simulink subsystem "ACS_Software"  (R2024a)
settings: Solver=VariableStepAuto  StartTime=0.0  StopTime=10.0  RelTol=1e-3
undefined symbols (not defined in the file): epoch, IAU, juliandate, k_Bdot, Kd, km, Kp, m, NoiseStd, s, signQuat, simulator, WMM2020
libraries: sharedtransform x15, simulink_extras x8, aerolibconvert2 x6, matrix_library x5, aerolibutil x5, aerolibtransform2 x2, sharedutil x1, SepehrMILLib x1, aerolibgravity2 x1
(part 2 of 2)

== system ACS_Software/Onboard Model of Environment/Reference Frames Transformations Manager/Quaternion Conditioner3 ==
  Q : Inport  PortDimensions=[4,1]
  Interpreted MATLAB Function : MATLABFcn  MATLABFcn=[u(1),0,0,0;0,u(2),0,0;0,0,u(3),0;0,0,0,u(4)]
  Interpreted MATLAB Function1 : MATLABFcn  MATLABFcn=[u(1),0,0,0;0,u(2),0,0;0,0,u(3),0;0,0,0,u(4)]
  Interpreted MATLAB Function2 : MATLABFcn  MATLABFcn=(u(1)+u(6)+u(11)+u(16))+1.9
  Product : Product
  Product1 : Product
  Sign : Signum
  Sign1 : Signum
  Unit Delay : UnitDelay  InitialCondition=[1;0;0;0]  SampleTime=-1  HasFrameUpgradeWarning=on
  Qc : Outport  PortDimensions=[4,1]
  wires:
  Unit Delay/1 -> Interpreted MATLAB Function1/1
  Interpreted MATLAB Function1/1 -> Product/2
  Q/1 -> Product1/1, Interpreted MATLAB Function/1
  Sign1/1 -> Product1/2
  Product/1 -> Sign/1
  Sign/1 -> Interpreted MATLAB Function2/1
  Interpreted MATLAB Function2/1 -> Sign1/1
  Interpreted MATLAB Function/1 -> Product/1
  Product1/1 -> Unit Delay/1, Qc/1

== system ACS_Software/Onboard Model of Environment/Reference Frames Transformations Manager/Quaternion Conditioner4 ==
  Q : Inport  PortDimensions=[4,1]
  Interpreted MATLAB Function : MATLABFcn  MATLABFcn=[u(1),0,0,0;0,u(2),0,0;0,0,u(3),0;0,0,0,u(4)]
  Interpreted MATLAB Function1 : MATLABFcn  MATLABFcn=[u(1),0,0,0;0,u(2),0,0;0,0,u(3),0;0,0,0,u(4)]
  Interpreted MATLAB Function2 : MATLABFcn  MATLABFcn=(u(1)+u(6)+u(11)+u(16))+1.9
  Product : Product
  Product1 : Product
  Sign : Signum
  Sign1 : Signum
  Unit Delay : UnitDelay  InitialCondition=[1;0;0;0]  SampleTime=-1  HasFrameUpgradeWarning=on
  Qc : Outport  PortDimensions=[4,1]
  wires:
  Product1/1 -> Qc/1, Unit Delay/1
  Interpreted MATLAB Function/1 -> Product/1
  Interpreted MATLAB Function2/1 -> Sign1/1
  Sign/1 -> Interpreted MATLAB Function2/1
  Product/1 -> Sign/1
  Sign1/1 -> Product1/2
  Q/1 -> Interpreted MATLAB Function/1, Product1/1
  Interpreted MATLAB Function1/1 -> Product/2
  Unit Delay/1 -> Interpreted MATLAB Function1/1

== matlab function ACS_Software/Attitude Determination and Estimation Algorithms/Quaternion Conditioner/MATLAB Function ==
  data: Diag_q input; y output
function y = fcn(Diag_q)

y = diag(Diag_q);

== matlab function ACS_Software/Attitude Determination and Estimation Algorithms/Quaternion Conditioner/MATLAB Function1 ==
  data: Diag_q input; y output
function y = fcn(Diag_q)

y = diag(Diag_q);

== stateflow chart ACS_Software/Attitude Control Algorithms1 ==
  state Detumbling
  state Transition
    entry: System_Mode;
  state Off
  state Nadir_Pointing
  Transition -> Detumbling [order 2] : [System_Mode == 1]
  (default) -> Transition
  Transition -> Off [order 3] : [System_Mode == 0]
  Transition -> Nadir_Pointing [order 1] : [System_Mode == 2]
  data: sf_internal_action_state_placeholder_data local double size=1 =0; sf_internal_action_state_placeholder_data local double size=1 =0; sf_internal_action_state_placeholder_data local double size=1 =0; System_Mode input; ACS_Command output; Sensors_Data input; Body2Orbit_Quaternions input; Direct_Commanded_Torque output

== matlab function ACS_Software/Attitude Determination and Estimation Algorithms/MATLAB Function10 ==
  data: u input; y output
function y = fcn(u)
% y=zeros(1);
if sum(isnan(u))>0
    disp('nan');
end
y = u;
end

== matlab function ACS_Software/Attitude Determination and Estimation Algorithms/MATLAB Function12 ==
  data: u input; y output
function y = fcn(u)
% y=zeros(1);
if sum(isnan(u))>0
    disp('nan');
end
y = u;
end

== matlab function ACS_Software/Attitude Determination and Estimation Algorithms/Normalizer4/NaNProtection ==
  data: u input; y output
function y = fcn(u)
lim = 1e-12;
if u < lim
    y = lim;
else
    y = u;
end

== matlab function ACS_Software/Attitude Determination and Estimation Algorithms/Quaternion Conditioner1/MATLAB Function1 ==
  data: Diag_q input; y output
function y = fcn(Diag_q)

y = diag(Diag_q);

== matlab function ACS_Software/Attitude Determination and Estimation Algorithms/Quaternion Conditioner1/MATLAB Function2 ==
  data: u input; y output
function y = fcn(u)
% y=zeros(1);
if sum(isnan(u))>0
    disp('nan');
end
y = (u(1)+u(6)+u(11)+u(16))+1.9;
end

== matlab function ACS_Software/Attitude Determination and Estimation Algorithms/MATLAB Function1 ==
  data: SunPos_ECI input; quat_TRIAD output; MagField_ECI input; SunPos_Body input; MagField_Body input; CovarianceMatrix output; RotationMatrix output; NoiseStd input; signQuat input
function [quat_TRIAD, CovarianceMatrix, RotationMatrix] = TRIAD(SunPos_ECI, MagField_ECI, SunPos_Body, MagField_Body, NoiseStd, signQuat)
% TRIAD Algorithm for Attitude Determination
% Inputs:
% - SunPos_ECI: Sun position vector in the inertial frame (ECI)
% - MagField_ECI: Magnetic field vector in the inertial frame (ECI)
% - SunPos_Body: Sun position vector in the body (spacecraft) frame
% - MagField_Body: Magnetic field vector in the body (spacecraft) frame
% - NoiseStd: [sigma1, sigma2] standard deviations of measurement noise
% - signQuat: sign parameter for quaternion calculation (e.g., ±1)
%
% Outputs:
% - quat_TRIAD: Quaternion representing the body-to-inertial rotation
% - CovarianceMatrix: Covariance matrix for the attitude estimation
% - RotationMatrix: Direction Cosine Matrix (DCM) from body to inertial frame

% Separate the noise standard deviations for more accurate and less accurate measurements
sigma_Sun = NoiseStd(1); % Standard deviation for Sun position measurement
sigma_Mag = NoiseStd(2); % Standard deviation for magnetic field measurement

% Reference Frame TRIAD Vectors (in ECI)
ref1 = SunPos_ECI;    % First vector (higher accuracy) in inertial frame
ref2 = cross(SunPos_ECI, MagField_ECI) / norm(cross(SunPos_ECI, MagField_ECI));
ref3 = cross(SunPos_ECI, ref2);  % Complete orthogonal basis

RefFrameMatrix = [ref1, ref2, ref3]; % TRIAD frame in terms of ECI vectors

% Body Frame TRIAD Vectors (in Spacecraft Frame)
body1 = SunPos_Body;  % First vector (higher accuracy) in body frame
body2 = cross(SunPos_Body, MagField_Body) / norm(cross(SunPos_Body, MagField_Body));
body3 = cross(SunPos_Body, body2); % Complete orthogonal basis

BodyFrameMatrix = [body1, body2, body3]; % TRIAD frame in terms of body vectors

% Estimated Rotation Matrix (DCM) from Body to Inertial Frame
RotationMatrix = RefFrameMatrix * BodyFrameMatrix';
RotationMatrix = transpose(RotationMatrix); % Transpose if convention requires it

% Convert Rotation Matrix to Quaternion
quat_TRIAD = DCMtoQuaternionLocal(RotationMatrix, signQuat);

% Covariance Matrix Calculation for TRIAD
CovarianceMatrix = 0;
% CovarianceMatrix = (sigma_Sun^2 * eye(3)) + ...
%     (((sigma_Mag^2 - sigma_Sun^2) * (body1 * body1')) + ...
%     (sigma_Sun^2 * (dot(body1, body2) * ((body1 * body2') + (body2 * body1'))))) / ...
%     (norm(cross(body1, body2))^2));

end

% Helper Function: DCM to Quaternion Conversion
function q = DCMtoQuaternionLocal(R, signQuat)
% Converts a Direction Cosine Matrix (DCM) to a Quaternion.
% Inputs:
% - R: Rotation matrix (3x3)
% - signQuat: Sign parameter for quaternion (e.g., ±1)
%
% Output:
% - q: Quaternion [q0; q1; q2; q3] where q0 is the scalar part

% Preallocate quaternion
q = zeros(4, 1);

% Calculate trace of the rotation matrix
traceR = trace(R);

if traceR > 0
    % Positive trace case
    S = sqrt(traceR + 1.0) * 2; % S=4*q0
    q(1) = 0.25 * S;            % q0
    q(2) = (R(3, 2) - R(2, 3)) / S; % q1
    q(3) = (R(1, 3) - R(3, 1)) / S; % q2
    q(4) = (R(2, 1) - R(1, 2)) / S; % q3
else
    % Trace is not positive
    if (R(1, 1) > R(2, 2)) && (R(1, 1) > R(3, 3))
        % R(1,1) is largest diagonal element
        S = sqrt(1.0 + R(1, 1) - R(2, 2) - R(3, 3)) * 2; % S=4*q1
        q(1) = (R(3, 2) - R(2, 3)) / S; % q0
        q(2) = 0.25 * S;               % q1
        q(3) = (R(1, 2) + R(2, 1)) / S; % q2
        q(4) = (R(1, 3) + R(3, 1)) / S; % q3
    elseif R(2, 2) > R(3, 3)
        % R(2,2) is largest
        S = sqrt(1.0 + R(2, 2) - R(1, 1) - R(3, 3)) * 2; % S=4*q2
        q(1) = (R(1, 3) - R(3, 1)) / S; % q0
        q(2) = (R(1, 2) + R(2, 1)) / S; % q1
        q(3) = 0.25 * S;               % q2
        q(4) = (R(2, 3) + R(3, 2)) / S; % q3
    else
        % R(3,3) is largest
        S = sqrt(1.0 + R(3, 3) - R(1, 1) - R(2, 2)) * 2; % S=4*q3
        q(1) = (R(2, 1) - R(1, 2)) / S; % q0
        q(2) = (R(1, 3) + R(3, 1)) / S; % q1
        q(3) = (R(2, 3) + R(3, 2)) / S; % q2
        q(4) = 0.25 * S;               % q3
    end
end

% Adjust sign if needed
q = signQuat * q;

end

== matlab function ACS_Software/Attitude Determination and Estimation Algorithms/MATLAB Function ==
  data: Sun_Vector_Body input; qTRIAD_Body2ICRF output; MagneticField_Body input; Sun_Vector_ICRF input; MagneticField_ICRF input
function qTRIAD_Body2ICRF = TRIAD(Sun_Vector_Body, MagneticField_Body, Sun_Vector_ICRF, MagneticField_ICRF)
    % TRIAD Algorithm to compute body-to-ICRF quaternion
    % Inputs:
    %   Sun_Vector_Body: Sun vector in the body frame (3x1)
    %   MagneticField_Body: Magnetic field vector in the body frame (3x1)
    %   Sun_Vector_ICRF: Sun vector in the ICRF frame (3x1)
    %   MagneticField_ICRF: Magnetic field vector in the ICRF frame (3x1)
    % Output:
    %   q_b2i: Quaternion (4x1) representing rotation from Body to ICRF frame

    % Normalize input vectors
    Sun_Vector_Body = Sun_Vector_Body / norm(Sun_Vector_Body);
    MagneticField_Body = MagneticField_Body / norm(MagneticField_Body);
    Sun_Vector_ICRF = Sun_Vector_ICRF / norm(Sun_Vector_ICRF);
    MagneticField_ICRF = MagneticField_ICRF / norm(MagneticField_ICRF);

    % Construct TRIAD basis in the Body frame
    t1_b = Sun_Vector_Body; % Primary vector
    t2_b = cross(Sun_Vector_Body, MagneticField_Body); % Secondary vector
    t2_b = t2_b / norm(t2_b); % Normalize secondary vector
    t3_b = cross(t1_b, t2_b); % Tertiary vector (orthogonal to t1_b and t2_b)

    % Construct TRIAD basis in the ICRF frame
    t1_i = Sun_Vector_ICRF; % Primary vector
    t2_i = cross(Sun_Vector_ICRF, MagneticField_ICRF); % Secondary vector
    t2_i = t2_i / norm(t2_i); % Normalize secondary vector
    t3_i = cross(t1_i, t2_i); % Tertiary vector (orthogonal to t1_i and t2_i)

    % Build rotation matrix from Body to ICRF frame
    R_b2i = [t1_i, t2_i, t3_i] * [t1_b, t2_b, t3_b]';

    % Convert rotation matrix to quaternion (ICRF to Body)
    qTRIAD_Body2ICRF = rotm2quat(R_b2i); % MATLAB's built-in function

    % Ensure quaternion is normalized
    qTRIAD_Body2ICRF = qTRIAD_Body2ICRF / norm(qTRIAD_Body2ICRF);
end

== matlab function ACS_Software/Attitude Determination and Estimation Algorithms/MATLAB Function2 ==
  data: obsSet input; quatSet output; refSet input; eulerSet output
function [quatSet, eulerSet] = TRIAD(obsSet,refSet)
%%% TRIAD Algorithm
%
% Inputs:
%   obsSet = Unit measurement vectors (3xn)
%   refSet = Unit reference vectors (3xn)
%
% Outputs:
%   quatSet = Quaternion set in body frame
%
% Reference:
%   [1] M. D. Shuster and S. D. Oh, Three-Axis Attitude Determination from
%       Vector Observations (1981)
%   [2] C. Hajiyev and H. E. Soken, Fault Tolerant Attitude Estimation for 
%       Small Satellites (2021), pp. 67-73
%
% Last Update: 8/8/2022 9:32 PM
    
    % Decompose observation and reference unit vectors where w_1 has the
    % greater accuracy
    v1 = refSet(:,1);
    v2 = refSet(:,2);
    w1 = obsSet(:,1);
    w2 = obsSet(:,2);

    % [1] Construct two triads [Eqs. (4) and (5)]
    r1 = v1;
    r2 = cross(v1,v2)/norm(cross(v1,v2));
    r3 = cross(v1,cross(v1,v2))/norm(cross(v1,v2));

    s1 = w1;
    s2 = cross(w1,w2)/norm(cross(w1,w2));
    s3 = cross(w1,cross(w1,w2))/norm(cross(w1,w2));

    % [1] Compose reference and body matrices [Eq. (9)]
    M_ref = [r1,r2,r3];
    M_obs = [s1,s2,s3];

    % [1] Compute the DCM (attitude matrix) [Eq. (8)]
    DCM = M_obs*M_ref';

    % [2] Build four 4-component vectors using the DCM, find the quaternion  
    % set by normalizing the most suitable component to reduce numerical 
    % errors [Eqs. (5.14a) and (5.14b)] 
    first =  [1+2*DCM(1,1)-trace(DCM);DCM(1,2)+DCM(2,1);
                    DCM(1,3)+DCM(3,1);DCM(2,3)-DCM(3,2)];

    second = [DCM(2,1)+DCM(1,2);1+2*DCM(2,2)-trace(DCM);
                    DCM(2,3)+DCM(3,2);DCM(3,1)-DCM(1,3)]; 

    third =  [DCM(1,3)+DCM(3,1);DCM(2,3)+DCM(3,2);
              1+2*DCM(3,3)-trace(DCM);DCM(1,2)-DCM(2,1)];

    fourth = [DCM(2,3)-DCM(3,2);DCM(3,1)-DCM(1,3);
                   DCM(1,2)-DCM(2,1);1+trace(DCM)];

    if DCM(1,1) == max([DCM(1,1),DCM(2,2),DCM(3,3),trace(DCM)])
        quatSet = first/norm(first);        
    elseif DCM(2,2) == max([DCM(1,1),DCM(2,2),DCM(3,3),trace(DCM)])
        quatSet = second/norm(second);
    elseif DCM(3,3) == max([DCM(1,1),DCM(2,2),DCM(3,3),trace(DCM)])
        quatSet = third/norm(third);
    elseif trace(DCM) == max([DCM(1,1),DCM(2,2),DCM(3,3),trace(DCM)])
        quatSet = fourth/norm(fourth);
    end 

    % Solution for Euler angles [Eq. (5.12)]
    eulerSet = [atan2(DCM(2,3),DCM(3,3));
                atan2(-DCM(1,3),sqrt(DCM(2,3)^2+DCM(3,3)^2));
                atan2(DCM(1,2),DCM(1,1))];
    
end

== matlab function ACS_Software/Attitude Determination and Estimation Algorithms/Quaternion Conditioner/MATLAB Function2 ==
  data: u input; y output
function y = fcn(u)
% y=zeros(1);
if sum(isnan(u))>0
    disp('nan');
end
y = (u(1)+u(6)+u(11)+u(16))+1.9;
end

== matlab function ACS_Software/Attitude Determination and Estimation Algorithms/Quaternion Conditioner1/MATLAB Function ==
  data: Diag_q input; y output
function y = fcn(Diag_q)

y = diag(Diag_q);

== matlab function ACS_Software/Attitude Control Algorithms1/Nadir_Pointing/Nadir Pointing Algorithm/PD Quaternion Feedback Controller/Dipole Smoother ==
  data: B input; m output; T_c input; k input
function m = computeMagneticDipole(B, T_c, k)
    % Computes the magnetic dipole moment (m) given:
    % B: Geomagnetic field vector in body frame [3x1] (T)
    % Tc: Commanded control torque in body frame [3x1] (N·m)
    % k: Regularization constant (scalar)
    %
    % Output:
    % m: Magnetic dipole moment in body frame [3x1] (A·m^2)

    % Validate inputs
    if length(B) ~= 3 || length(T_c) ~= 3
        error('B and Tc must be 3x1 vectors.');
    end

    % Create the skew-symmetric matrix of B
    B_mat = [
        0,       B(3),  -B(2);
       -B(3),   0,       B(1);
        B(2),  -B(1),    0
    ];

    % Compute the SR-Inverse
    I = eye(3); % 3x3 identity matrix
    regularized_inverse = inv((B_mat.' * B_mat + k * I)) / B_mat.';

    % Compute the magnetic dipole moment
    m = regularized_inverse * T_c;
end

== matlab function ACS_Software/Attitude Determination and Estimation Algorithms/MATLAB Function3 ==
  data: v1_B input; A_BI output; v1_I input; v2_B input; v2_I input
function A_BI  = triad(v1_B, v1_I, v2_B, v2_I)
%TRIAD Implements the triad algorithm to calculate a direction cosine
%matrix (DCM) representing the rotation of the body frame relative to the
%inertial frame. (See textbook section 5.1)
%   This function accepts 2 vectors both in the body and inertial frames,
%   prioritizing the first vector measurements and returns the calculated
%   DCM. It is implemented as in Equation 5.6
u1_B = v1_B/norm(v1_B);
u1_I = v1_I/norm(v1_I);

u2_B = cross(u1_B, v2_B);
u2_B = u2_B/norm(u2_B);
u2_I = cross(u1_I,v2_I);
u2_I = u2_I/norm(u2_I);

u3_B = cross(u1_B, u2_B);
u3_I = cross(u1_I, u2_I);

A_BI = u1_B*u1_I' + u2_B*u2_I' + u3_B*u3_I';
end
